simulink library "gravity_gradient"  (R2020b)
settings: Solver=VariableStepAuto  StartTime=0.0  StopTime=10.0  RelTol=1e-3
settings Model: Creator=whitehole  LastModifiedBy=whitehole

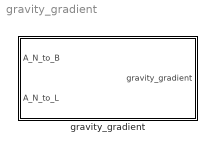
== system gravity_gradient ==
  gravity_gradient : Subsystem

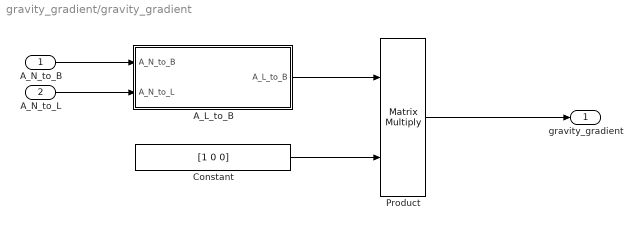
== system gravity_gradient/gravity_gradient ==
  A_N_to_B : Inport
  A_N_to_L : Inport  Port=2
  A_L_to_B : Subsystem
  Constant : Constant  Value=[1 0 0]
  Product : Product  Multiplication=Matrix(*)
  gravity_gradient : Outport
  wires:
  A_N_to_L/1 -> A_L_to_B/2(A_N_to_L)
  Constant/1 -> Product/2
  A_N_to_B/1 -> A_L_to_B/1(A_N_to_B)
  Product/1 -> gravity_gradient/1
  A_L_to_B/1(A_L_to_B) -> Product/1

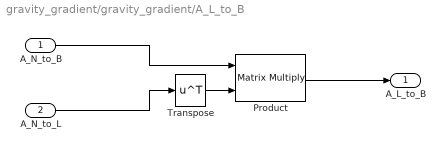
== system gravity_gradient/gravity_gradient/A_L_to_B ==
  A_N_to_B : Inport
  A_N_to_L : Inport  Port=2
  Product : Product  Multiplication=Matrix(*)
  Transpose : Math  Operator=transpose  SaturateOnIntegerOverflow=on
  A_L_to_B : Outport
  wires:
  A_N_to_L/1 -> Transpose/1
  Product/1 -> A_L_to_B/1
  Transpose/1 -> Product/2
  A_N_to_B/1 -> Product/1
